simulink model "WK_MaoBi_09102013_Offline"  (Simulink 7.7)
settings: Solver=ode4  StartTime=0.0  StopTime=inf  FixedStep=sample_time  RelTol=1e-3
InitFcn:
  | sample_time=0.005;%0.004;%0.0025;%0.02;
  | DeltaT = 0.02;
  | g = 9.81;
  | H0 = g%0.3165;
  | Kl = 1;
  | 
  | Omega_r = 1.6;%for Horizontal reference
  | Zeta_r = 0.7; %for Horizontal reference
  | Omega = 1.8;%for Horizontal Control
  | Zeta = 0.5;    %for Horizontal Control
  | 
  | Omega_h_r = 2.5; %for vertical reference
  | Zeta_h_r = 0.8;  %for vertical reference
  | Omega_h = 2.7;    %for vertical control
  | Zeta_h = 0.8;         %for vertical control
  | PI=pi;
  | 
  | Mass = 1.1;
  | Acc_Max = 4;
  | Acc_Max_h = 4;
  | 
  | Max_RP = 60;
  | 
  | load MaoBi_Oct04_2_int.mat
  | MB_Interp.time = [];
undefined symbols (not defined in the file or in its folder): DiscIntNeverNeededParam
libraries: simulink x7, dspadpt3 x3, X330_Control x2, X400_Control x1
(part 2 of 2)

== stateflow chart Planning/Trajectory Logic/UAV SF ==
  state Landing
    state Descending
      en:PosDesired = Pos;
      du:PosDesired[2] = (PerchPos[2]- PosDesired[2])*1*DeltaT + PosDesired[2] ;
    state CutThrottle
      du:HoverThrottle = (0 - HoverThrottle)*3*DeltaT + HoverThrottle ;
    (default) -> Descending
    Descending -> CutThrottle : [Pos[2] > (PerchPos[2]-0.1)]
  state Airborne
    state TakeOff
      du:HoverThrottle = (H0 - HoverThrottle)*3*DeltaT + HoverThrottle ;
    state MB3
      en:
      PosDesired[0]=-1.0, PosDesired[1]=1.23;
    state MB2
      en:
      PosDesired[0]=-1.0, PosDesired[1]=1.23,PosDesired[2]=-0.7;
    state SafyHover
      en:PosDesired = Pos; PosDesired[2]=-1.2;
    state Prelanding
      en:PosDesired[0] = PerchPos[0]; PosDesired[1] = PerchPos[1];PosDesired[2] = PerchPos[2]-0.5 ;
    state Descent
      en:PosDesired[2] = PerchPos[2]-0.2;
    state MB
      en:
      PosDesired[0]=-1.0, PosDesired[1]=1.0,PosDesired[2]=-0.8;
    state SafyHover1
      en:PosDesired = Pos; PosDesired[2]=-1.2;
    state MB4
      en:
      PosDesired[0]=-1.23, PosDesired[1]=1.23,PosDesired[2]=-0.7;
    state MB5
      en:
      PosDesired[0]=-1.23, PosDesired[1]=1.23;
    state MB6
      en:
      PosDesired[0]=-1.23, PosDesired[1]=1.0,PosDesired[2]=-0.7;
    state MB7
      en:
      PosDesired[0]=-1.23, PosDesired[1]=1.0;
    state MB8
      en:
      PosDesired[0]=-1.0, PosDesired[1]=1.0,PosDesired[2]=-0.7;
    state MB9
      en:
      PosDesired[0]=-1.23, PosDesired[1]=1.0;
    state Descent1
      en:PosDesired[2] = PerchPos[2]-0.1;
    state Brushdown
      en:
      PosDesired[0] = -1.0; PosDesired[1] = 1.0;PosDesired[2]=-0.7;
    state Brushup
      en:
      PosDesired[0]=-1.0;PosDesired[1]=1.23;PosDesired[2]=-0.75;
    state Brushdown1
      en:
      PosDesired[0]=-1.0;PosDesired[1]=1.23;PosDesired[2]=-0.7;
    state Brushup2
      en:
      PosDesired[0]=-1.23;PosDesired[1]=1.23;PosDesired[2]=-0.75;
    state Brushup3
      en:
      PosDesired[0]=-1.23;PosDesired[1]=1.0;PosDesired[2]=-0.75;
    state Brushdown2
      en:
      PosDesired[0]=-1.23;PosDesired[1]=1.23;PosDesired[2]=-0.7;
    state Brushdown3
      en:
      Posdesired[0]=-1.23;PosDesired[1]=1.0;PosDesired[2]=-0.7;
    state Brushup4
      en:
      PosDesired[0]=-1.0;PosDesired[1]=1.0;PosDesired[2]=-0.75;
    state Brushdown4
      en:
      PosDesired[0]=-1.23;PosDesired[1]=1.0;PosDesired[2]=-0.65;
    state MB10
      en:
      PosDesired[0]=-1.0, PosDesired[1]=1.23, PosDesired[2] = -0.65;
    state Brushup5
      en:
      PosDesired[2]=-0.9;
    Brushup4 -> SafyHover1 [order 1] : [RC[5] > 0]
    MB3 -> SafyHover [order 2] : [RC[5] > 0]
    TakeOff -> MB : after(5,sec)
    SafyHover -> Prelanding : after (3, sec)
    Prelanding -> Descent : [PerchError < 0.01]
    Brushup5 -> SafyHover1 : [RC[5] > 0]
    MB2 -> Brushup [order 1] : [abs(PosDesired[0]-Pos[0])+abs(PosDesired[1]-Pos[1])+abs(PosDesired[2]-Pos[2])<0.03]
    MB -> Brushdown [order 1] : [abs(PosDesired[0]-Pos[0])+abs(PosDesired[1]-Pos[1])<0.01]
    MB -> SafyHover [order 2] : [RC[5] > 0]
    Brushdown4 -> SafyHover1 [order 1] : [RC[5] > 0]
    MB2 -> SafyHover [order 2] : [RC[5] > 0]
    Brushdown1 -> MB4 [order 2] : [abs(PosDesired[2]-Pos[2])<0.01]
    MB4 -> SafyHover [order 2] : [RC[5] > 0]
    Brushup2 -> MB5 [order 2] : [abs(PosDesired[2]-Pos[2])<0.01]
    MB5 -> Brushdown2 [order 1] : [abs(PosDesired[0]-Pos[0])+abs(PosDesired[1]-Pos[1])<0.01]
    MB6 -> Brushup3 [order 1] : [abs(PosDesired[0]-Pos[0])+abs(PosDesired[1]-Pos[1])+abs(PosDesired[2]-Pos[2])<0.03]
    Brushdown3 -> MB8 [order 2] : [abs(PosDesired[2]-Pos[2])<0.01]
    MB8 -> Brushup4 [order 1] : [abs(PosDesired[0]-Pos[0])+abs(PosDesired[1]-Pos[1])+abs(PosDesired[2]-Pos[2])<0.03]
    MB5 -> SafyHover [order 2] : [RC[5] > 0]
    MB6 -> SafyHover [order 2] : [RC[5] > 0]
    MB7 -> SafyHover [order 2] : [RC[5] > 0]
    MB8 -> SafyHover [order 2] : [RC[5] > 0]
    MB9 -> SafyHover [order 2] : [RC[5] > 0]
    Descent -> Descent1 [order 2] : [PerchError < 0.01]
    Brushdown -> MB2 [order 2] : [abs(PosDesired[2]-Pos[2])<0.01]
    Brushup -> MB3 [order 2] : [abs(PosDesired[2]-Pos[2])<0.01]
    MB3 -> Brushdown1 [order 1] : [abs(PosDesired[0]-Pos[0])+abs(PosDesired[1]-Pos[1])<0.01]
    MB4 -> Brushup2 [order 1] : [abs(PosDesired[0]-Pos[0])+abs(PosDesired[1]-Pos[1])+abs(PosDesired[2]-Pos[2])<0.03]
    Brushdown2 -> MB6 [order 2] : [abs(PosDesired[2]-Pos[2])<0.01]
    Brushup3 -> MB7 [order 2] : [abs(PosDesired[2]-Pos[2])<0.01]
    (default) -> TakeOff : {PosDesired = Pos;  PosDesired[2] =-1.2;}
    Brushup4 -> MB9 [order 2] : [abs(PosDesired[2]-Pos[2])<0.01]
    MB9 -> Brushdown4 [order 1] : [abs(PosDesired[0]-Pos[0])+abs(PosDesired[1]-Pos[1])<0.01]
    Brushdown4 -> MB10 [order 2] : [abs(PosDesired[2]-Pos[2])<0.01]
    MB10 -> Brushup5 [order 1] : [abs(PosDesired[0]-Pos[0])+abs(PosDesired[1]-Pos[1])+abs(PosDesired[2]-Pos[2])<0.03]
    MB10 -> SafyHover [order 2] : [RC[5] > 0]
    Brushdown -> SafyHover1 [order 1] : [RC[5] > 0]
    Brushup -> SafyHover1 [order 1] : [RC[5] > 0]
    Brushdown1 -> SafyHover1 [order 1] : [RC[5] > 0]
    Brushup2 -> SafyHover1 [order 1] : [RC[5] > 0]
    Brushdown2 -> SafyHover1 [order 1] : [RC[5] > 0]
    Brushup3 -> SafyHover1 [order 1] : [RC[5] > 0]
    Brushdown3 -> SafyHover1 [order 1] : [RC[5] > 0]
    MB7 -> Brushdown3 [order 1] : [abs(PosDesired[0]-Pos[0])+abs(PosDesired[1]-Pos[1])<0.01]
    Descent1 -> Prelanding : after (6,sec)
    Descent -> Prelanding [order 1] : after (6,sec)
  (default) -> Landing : {HoverThrottle = 0;}
  Airborne -> Landing : [RC[6] < -0.5]
  Landing -> Airborne : [RC[6] > 0.5]
  SafyHover1 -> Prelanding : after (3, sec)
  data: PosDesired output double size=4; HoverThrottle output double size=1; Mode output uint8 size=1; RC input double size=8; Pos input double size=4; PerchPos input double size=4; DeltaT parameter double size=1; H0 parameter double size=1; Kl parameter double size=1; VelCmd local double size=2 =0; PWM output double; PerchError input double; PI parameter double size=1; Brush input double size=3; Check local double
